simulink model "LUT"  (R2022a)
settings: Solver=VariableStepAuto  StartTime=0.0  StopTime=10.0  RelTol=1e-3
settings Model: Creator=Ruwinda Nanayakkara  LastModifiedBy=Ruwinda Nanayakkara

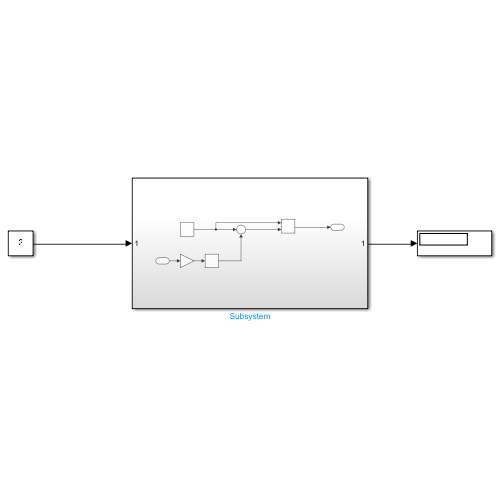
[thumbnail: Simulink's stored preview of the top-level diagram]
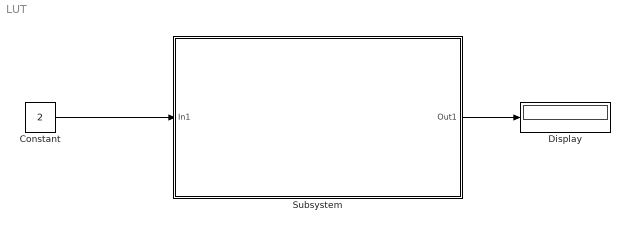
== system LUT ==
  Constant : Constant  Value=2
  Display : Display
  Subsystem : Subsystem
  wires:
  Constant/1 -> Subsystem/1(In1)
  Subsystem/1(Out1) -> Display/1

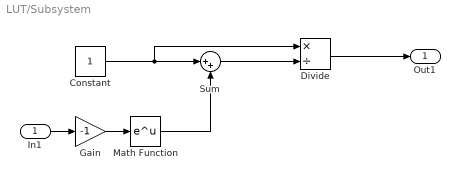
== system LUT/Subsystem ==
  In1 : Inport
  Constant : Constant
  Divide : Product  Inputs=*/
  Gain : Gain  Gain=-1
  Math Function : Math
  Sum : Sum  Inputs=|++
  Out1 : Outport
  wires:
  In1/1 -> Gain/1
  Gain/1 -> Math Function/1
  Math Function/1 -> Sum/2
  Constant/1 -> Divide/1, Sum/1
  Sum/1 -> Divide/2
  Divide/1 -> Out1/1
